simulink model "cukConverter"  (R2021a)
settings: Solver=VariableStepAuto  StartTime=0.0  StopTime=0.1  RelTol=1e-3
libraries: spsSeriesRLCBranchLib x5, spsVoltageMeasurementLib x3, spsCurrentMeasurementLib x2, spsDiodeLib x1, spsMosfetLib x1, spsPWMGeneratorDCDCLib x1, spsDCVoltageSourceLib x1, spspowerguiLib x1
settings Model: Creator=ASUS  LastModifiedBy=ASUS

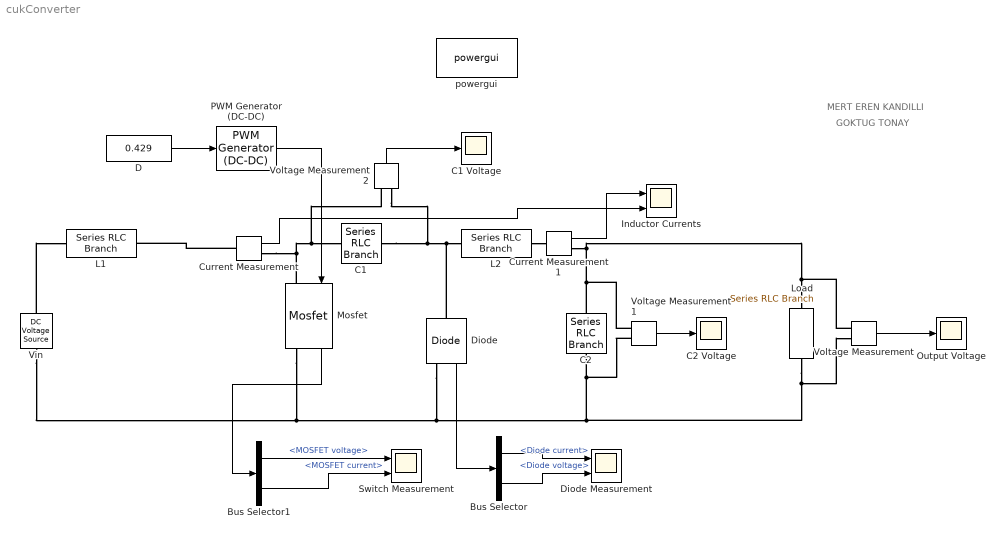
== system cukConverter ==
  note: GOKTUG TONAY
  note: MERT EREN KANDILLI
  Bus Selector : BusSelector  OutputSignals=Diode current,Diode voltage
  Bus Selector1 : BusSelector  OutputSignals=MOSFET voltage,MOSFET current
  C1 : spsSeriesRLCBranchLib/Series RLC Branch  LConnTagsString=__new0  RConnTagsString=__new0  BranchType=C  Resistance=1e-4  Inductance=200e-6  SetiL0=off  InitialCurrent=0  Capacitance=6.8e-6  Setx0=off  InitialVoltage=40  Measurements=None
  C1 Voltage : Scope
  C2 : spsSeriesRLCBranchLib/Series RLC Branch  LConnTagsString=__new0  RConnTagsString=__new0  BranchType=C  Resistance=1e-4  Inductance=200e-6  SetiL0=off  InitialCurrent=0  Capacitance=2.2e-6  Setx0=on  InitialVoltage=0  Measurements=None
  C2 Voltage : Scope
  Current Measurement : spsCurrentMeasurementLib/Current Measurement  PhasorSimulation=off  OutputType=Complex  PSBequivalent=0
  Current Measurement1 : spsCurrentMeasurementLib/Current Measurement  PhasorSimulation=off  OutputType=Complex  PSBequivalent=0
  D : Constant  Value=0.429
  Diode : spsDiodeLib/Diode  Ron=1e-3  Lon=0  Vf=0.4  IC=0  UseSnubber=off  Rs=inf  Cs=inf  Measurements=on
  Diode Measurement : Scope  NumInputPorts=2
  Inductor Currents : Scope  NumInputPorts=2
  L1 : spsSeriesRLCBranchLib/Series RLC Branch  LConnTagsString=__new0  RConnTagsString=__new0  BranchType=RL  Resistance=0.6  Inductance=1e-3  SetiL0=on  InitialCurrent=0  Capacitance=1e-6  Setx0=off  InitialVoltage=0  Measurements=Branch current
  L2 : spsSeriesRLCBranchLib/Series RLC Branch  LConnTagsString=__new0  RConnTagsString=__new0  BranchType=RL  Resistance=118e-3  Inductance=0.680e-3  SetiL0=on  InitialCurrent=0  Capacitance=1e-6  Setx0=off  InitialVoltage=0  Measurements=Branch current
  Load : spsSeriesRLCBranchLib/Series RLC Branch  LConnTagsString=__new0  RConnTagsString=__new0  BranchType=R  Resistance=6  Inductance=200e-6  SetiL0=off  InitialCurrent=0  Capacitance=400e-6  Setx0=off  InitialVoltage=0  Measurements=None
  Mosfet : spsMosfetLib/Mosfet  Ron=1e-3  Lon=0  Rd=1e-3  Vfd=24e-3  IC=0  Rs=1e6  Cs=inf  Measurements=on
  Output Voltage : Scope
  PWM Generator (DC-DC) : spsPWMGeneratorDCDCLib/PWM Generator (DC-DC)  Fsw=50e3  Ts=0
  Switch Measurement : Scope  NumInputPorts=2
  Vin : spsDCVoltageSourceLib/DC Voltage Source  Amplitude=16  Measurements=None
  Voltage Measurement : spsVoltageMeasurementLib/Voltage Measurement  PhasorSimulation=off  OutputType=Complex  PSBequivalent=0
  Voltage Measurement1 : spsVoltageMeasurementLib/Voltage Measurement  PhasorSimulation=off  OutputType=Complex  PSBequivalent=0
  Voltage Measurement2 : spsVoltageMeasurementLib/Voltage Measurement  PhasorSimulation=off  OutputType=Complex  PSBequivalent=0
  powergui : spspowerguiLib/powergui  Priority=1  SimulationMode=Continuous  SampleTime=50e-6  frequency=60  Iterations=50  frequencyindice=0  Pbase=100e6  ErrMax=1e-4  UnitsV=kV  UnitsW=MW  buscounter=0  FunctionMessages=off  echomessages=off  EnableUseOfTLC=off  CurrentSourceSwitches=off  DisableSnubberDevices=off  DisableRonSwitches=off  DisableVfSwitches=off  DisplayEquations=off  AutomaticDiscreteSolvers=off  SolverType=Tustin/Backward Euler (TBE)  Interpol=off  ExternalGateDelay=off  methode=off  Ts=10  x0status=blocks  SPID=on  SwTol=0  HookPort=off  NonlinearTolerance=1e-4  nMaxIteration=100  ContinueOnMaxIteration=off  RestoreLinks=warning  ResistiveCurrentMeasurement=off  Frange=[0:2:500]  Ylog=off  Xlog=on  ShowGrid=off  save=off  variable=ZData  structure=0  ZoomFFT=off  StartTime=0.0  cycles=1  DisplayStyle=1  fundamental=60  FreqAxis=off  MaxFrequency=1000  frequencyindicesteady=1  RmsSteady=1  display=off
  wires:
  Voltage Measurement1/1 -> C2 Voltage/1
  Diode/1 -> Bus Selector/1
  Bus Selector/2 -> Diode Measurement/2  "<Diode voltage>"
  Bus Selector/1 -> Diode Measurement/1  "<Diode current>"
  Bus Selector1/1 -> Switch Measurement/1  "<MOSFET voltage>"
  D/1 -> PWM Generator (DC-DC)/1
  PWM Generator (DC-DC)/1 -> Mosfet/1
  Voltage Measurement/1 -> Output Voltage/1
  Bus Selector1/2 -> Switch Measurement/2  "<MOSFET current>"
  Mosfet/1 -> Bus Selector1/1
  Voltage Measurement2/1 -> C1 Voltage/1
  Current Measurement/1 -> Inductor Currents/2
  Current Measurement1/1 -> Inductor Currents/1
  connections:
  C2/LConn1 -- Voltage Measurement1/LConn1 -- Voltage Measurement/LConn1 -- Load/LConn1 -- Current Measurement1/RConn1
  L2/LConn1 -- C1/RConn1 -- Voltage Measurement2/LConn2 -- Diode/LConn1
  Mosfet/LConn1 -- C1/LConn1 -- Voltage Measurement2/LConn1 -- Current Measurement/RConn1
  Diode/RConn1 -- Load/RConn1 -- Voltage Measurement/LConn2 -- Voltage Measurement1/LConn2 -- C2/RConn1 -- Mosfet/RConn1 -- Vin/LConn1
  Vin/RConn1 -- L1/LConn1
  Current Measurement/LConn1 -- L1/RConn1
  L2/RConn1 -- Current Measurement1/LConn1
